simulink model "rfsstudy"  (Simulink 5.0)
settings: Solver=ode23tb  StartTime=0.0  StopTime=inf  MaxStep=1/900000  MinStep=1/1000000000  RelTol=1e-6
undefined symbols (not defined in the file or in its folder): get, RFSSimple
libraries: simulink x2, commcontsrc2 x2, dspsnks4 x1
settings Model: LastModifiedBy=efst  SimulationMode=accelerator

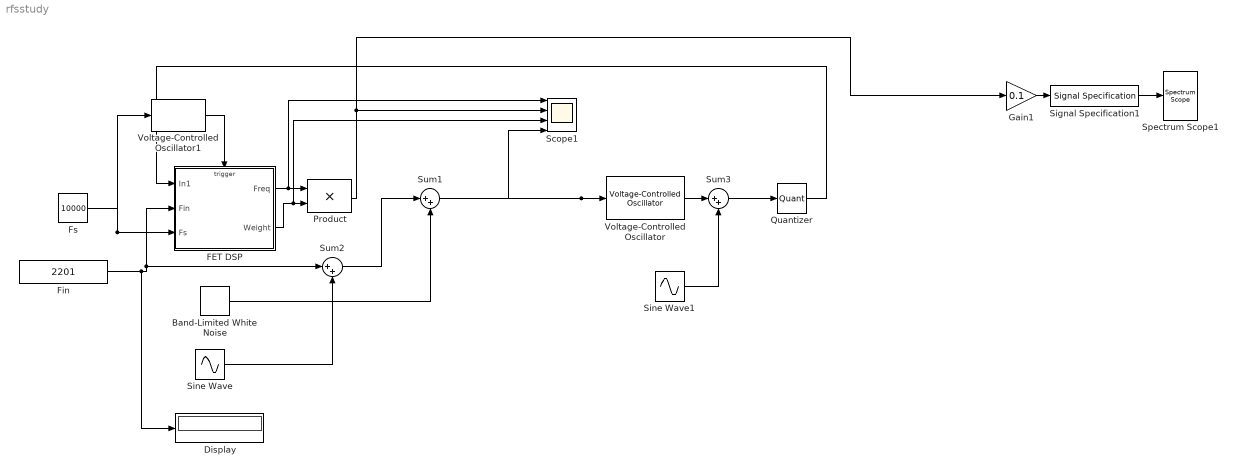
== system rfsstudy ==
  Band-Limited White Noise : simulink/Sources/Band-Limited White Noise  Cov=[0.00000]  Ts=1/10000  seed=[23341]
  Display : Display
  FET DSP : Subsystem  TreatAsAtomicUnit=on
  Fin : Constant  Value=2201
  Fs : Constant  Value=10000
  Gain1 : Gain  Gain=0.1  SaturateOnIntegerOverflow=on
  Product : Product  SaturateOnIntegerOverflow=on
  Quantizer : Quantizer  QuantizationInterval=2/(2^12)
  Scope1 : Scope  NumInputPorts=4
      settings: TimeRange=0.01  YMin=-10~-1.25~0~2201  YMax=25~1~1~2201
  Signal Specification1 : simulink/Signal Attributes/Signal Specification  D=1  Ts=1/10000  DataType=auto  OutDataType=sfix(16)  OutScaling=2^0
      settings: SignalType=auto  SamplingMode=sample-based
  Sine Wave : Sin  Amplitude=0.0  Frequency=2*pi*500  SampleTime=0
  Sine Wave1 : Sin  Amplitude=0.00  Frequency=2*pi*500  SampleTime=0
  Spectrum Scope1 : dspsnks4/Spectrum Scope  ScopeProperties=on  Domain=Frequency  HorizSpan=1  UseBuffer=on  BufferSize=2048  Overlap=64  inpFftLenInherit=on  FFTlength=2048  numAvg=2  DisplayProperties=off  AxisGrid=on  Memory=off  FrameNumber=on  AxisLegend=off  AxisZoom=off  OpenScopeAtSimStart=on  OpenScopeImmediately=off  FigPos=get(0,'defaultfigureposition')  AxisProperties=off  XUnits=Hertz  XRange=[0...Fs/2]  InheritXIncr=on  XIncr=1.0  XLabel=Samples  YUnits=dB  YLabel=Magnitude, dB  LineProperties=off
      settings: YMin=-67.4323242420501  YMax=4.28535562894144
  Sum1 : Sum  Inputs=|++  SaturateOnIntegerOverflow=on
  Sum2 : Sum  Inputs=|++  SaturateOnIntegerOverflow=on
  Sum3 : Sum  Inputs=|++  SaturateOnIntegerOverflow=on
  Voltage-Controlled Oscillator : commcontsrc2/Voltage-Controlled Oscillator  Ac=1  Fc=0  Kc=1  Ph=0
  Voltage-Controlled Oscillator1 : commcontsrc2/Voltage-Controlled Oscillator  Ac=1  Fc=0  Kc=1  Ph=0
  wires:
  Fs/1 -> FET DSP/3(Fs), Voltage-Controlled Oscillator1/1
  Voltage-Controlled Oscillator1/1 -> FET DSP/Trigger
  FET DSP/1(Freq) -> Product/1, Scope1/1
  FET DSP/2(Weight) -> Product/2, Scope1/3
  Fin/1 -> FET DSP/2(Fin), Sum2/1, Display/1
  Sum1/1 -> Voltage-Controlled Oscillator/1, Scope1/4
  Band-Limited White Noise/1 -> Sum1/2
  Product/1 -> Scope1/2, Gain1/1
  Quantizer/1 -> FET DSP/1(In1)
  Signal Specification1/1 -> Spectrum Scope1/1
  Gain1/1 -> Signal Specification1/1
  Sum2/1 -> Sum1/1
  Sine Wave/1 -> Sum2/2
  Voltage-Controlled Oscillator/1 -> Sum3/1
  Sum3/1 -> Quantizer/1
  Sine Wave1/1 -> Sum3/2

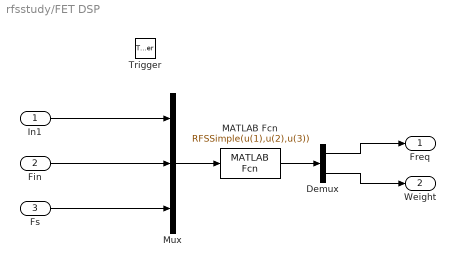
== system rfsstudy/FET DSP ==
  In1 : Inport
  Fin : Inport  Port=2
  Fs : Inport  Port=3
  Trigger : TriggerPort
  Demux : Demux  Outputs=2
  MATLAB Fcn : MATLABFcn  MATLABFcn=RFSSimple(u(1),u(2),u(3))  OutputDimensions=2  OutputSignalType=real  Output1D=off
  Mux : Mux  Inputs=3
  Freq : Outport
  Weight : Outport  Port=2
  wires:
  Fin/1 -> Mux/2
  Mux/1 -> MATLAB Fcn/1
  In1/1 -> Mux/1
  Fs/1 -> Mux/3
  MATLAB Fcn/1 -> Demux/1
  Demux/1 -> Freq/1
  Demux/2 -> Weight/1
